simulink library "ESTS_VSLARE"  (R2024b)
settings: Solver=VariableStepAuto  StartTime=0.0  StopTime=10.0  RelTol=1e-3
libraries: VUT_lib x3
settings Model: Creator=blatak  LastModifiedBy=blatak

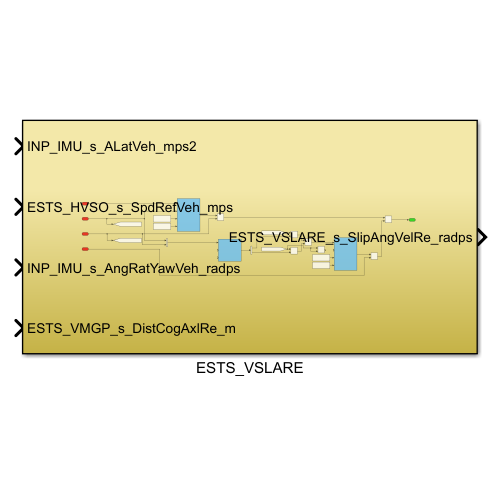
[thumbnail: Simulink's stored preview of the top-level diagram]
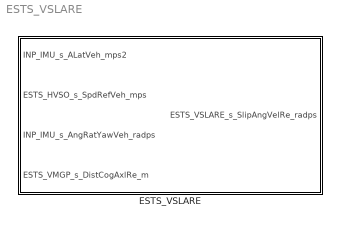
== system ESTS_VSLARE ==
  ESTS_VSLARE : Subsystem

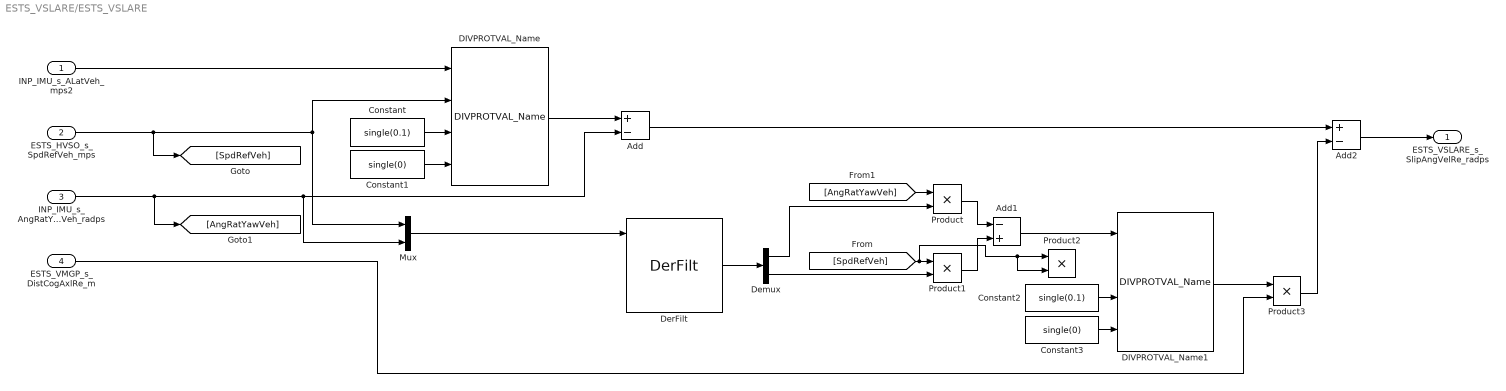
== system ESTS_VSLARE/ESTS_VSLARE ==
  INP_IMU_s_ALatVeh_mps2 : Inport
  ESTS_HVSO_s_SpdRefVeh_mps : Inport  Port=2
  INP_IMU_s_AngRatYawVeh_radps : Inport  Port=3
  ESTS_VMGP_s_DistCogAxlRe_m : Inport  Port=4
  Add : Sum  Inputs=+-
  Add1 : Sum  Inputs=-+
  Add2 : Sum  Inputs=+-
  Constant : Constant  Value=single(0.1)
  Constant1 : Constant  Value=single(0)
  Constant2 : Constant  Value=single(0.1)
  Constant3 : Constant  Value=single(0)
  DIVPROTVAL_Name : VUT_lib/DIVPROTVAL_Name  SystemSampleTime=-1  VariantActivationTime=update diagram  AllowFlexibleInterface=on  Latency=0  AutoFrameSizeCalculation=off
  DIVPROTVAL_Name1 : VUT_lib/DIVPROTVAL_Name  SystemSampleTime=-1  VariantActivationTime=update diagram  AllowFlexibleInterface=on  Latency=0  AutoFrameSizeCalculation=off
  Demux : Demux  Outputs=2
  DerFilt : VUT_lib/DerFilt  SystemSampleTime=-1  VariantActivationTime=update diagram  AllowFlexibleInterface=on  Latency=0  AutoFrameSizeCalculation=off
  Mux : Mux  Inputs=2
  Product{,1..3} (4 alike) : Product
  ESTS_VSLARE_s_SlipAngVelRe_radps : Outport
  wires:
  INP_IMU_s_ALatVeh_mps2/1 -> DIVPROTVAL_Name/1
  ESTS_HVSO_s_SpdRefVeh_mps/1 -> [SpdRefVeh], DIVPROTVAL_Name/2, Mux/1
  Constant/1 -> DIVPROTVAL_Name/3
  Constant1/1 -> DIVPROTVAL_Name/4
  DIVPROTVAL_Name/1 -> Add/1
  INP_IMU_s_AngRatYawVeh_radps/1 -> [AngRatYawVeh], Mux/2, Add/2
  Mux/1 -> DerFilt/1
  DerFilt/1 -> Demux/1
  Demux/2 -> Product1/2
  [SpdRefVeh] -> Product2/2, Product2/1, Product1/1
  Demux/1 -> Product/2
  [AngRatYawVeh] -> Product/1
  Product1/1 -> Add1/2
  Product/1 -> Add1/1
  Add1/1 -> DIVPROTVAL_Name1/1
  Constant2/1 -> DIVPROTVAL_Name1/3
  Constant3/1 -> DIVPROTVAL_Name1/4
  DIVPROTVAL_Name1/1 -> Product3/1
  ESTS_VMGP_s_DistCogAxlRe_m/1 -> Product3/2
  Product3/1 -> Add2/2
  Add/1 -> Add2/1
  Add2/1 -> ESTS_VSLARE_s_SlipAngVelRe_radps/1
